simulink model "test_RBFNN"  (R2019a)
settings: Solver=ode45  StartTime=0.0  StopTime=65  RelTol=1e-3
settings Model: Creator=huic  LastModifiedBy=huic

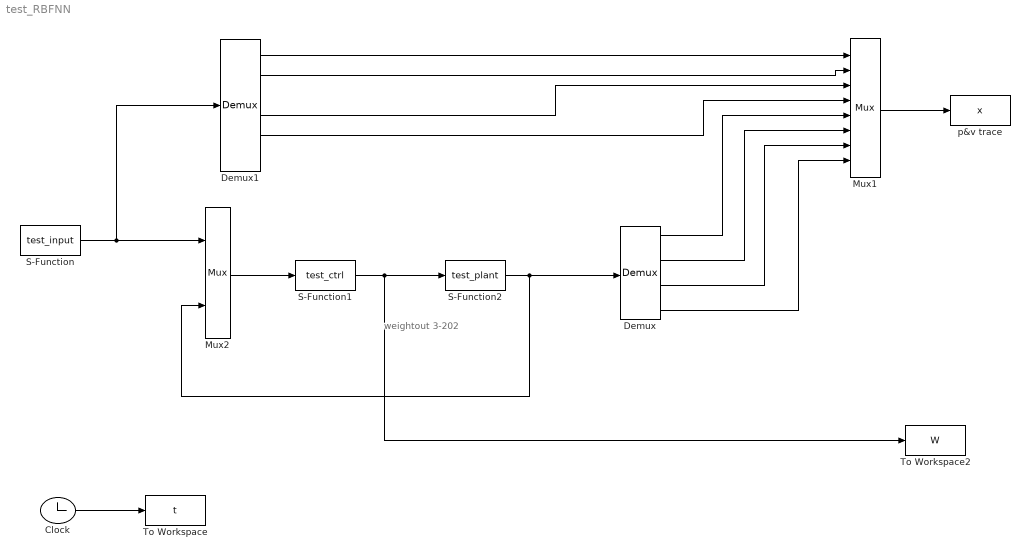
== system test_RBFNN ==
  note: weightout 3-202
  Clock : Clock
  Demux : Demux
  Demux1 : Demux  Outputs=6
  Mux1 : Mux  Inputs=8
  Mux2 : Mux  Inputs=2
  S-Function : S-Function  FunctionName=test_input  SFunctionDeploymentMode=off  EnableBusSupport=off
  S-Function1 : S-Function  FunctionName=test_ctrl  SFunctionDeploymentMode=off  EnableBusSupport=off
  S-Function2 : S-Function  FunctionName=test_plant  SFunctionDeploymentMode=off  EnableBusSupport=off
  To Workspace : ToWorkspace  VariableName=t  SampleTime=-1
  To Workspace2 : ToWorkspace  VariableName=W  SampleTime=-1
  p&v trace : ToWorkspace  VariableName=x  SampleTime=-1
  wires:
  S-Function1/1 -> To Workspace2/1, S-Function2/1
  S-Function2/1 -> Mux2/2, Demux/1
  S-Function/1 -> Demux1/1, Mux2/1
  Mux2/1 -> S-Function1/1
  Demux1/1 -> Mux1/1
  Demux/1 -> Mux1/5
  Clock/1 -> To Workspace/1
  Mux1/1 -> p&v trace/1
  Demux1/2 -> Mux1/2
  Demux1/4 -> Mux1/3
  Demux1/5 -> Mux1/4
  Demux/2 -> Mux1/6
  Demux/3 -> Mux1/7
  Demux/4 -> Mux1/8
